simulink model "Linear_wReduced_Observer"  (R2022a)
settings: Solver=VariableStepAuto  StartTime=0.16733  StopTime=3000.0185  RelTol=1e-3
undefined symbols (not defined in the file): A_HD, A_platform, B_HD, B_platform, C_HD, C_platform, HD_FOP
settings Model: Creator=ianam  LastModifiedBy=ianam
settings DataIOCC: InitialState=IC  LoadInitialState=on
settings DebuggingCC: UnderSpecifiedDataTypeMsg=error  UnderSpecifiedDimensionMsg=error

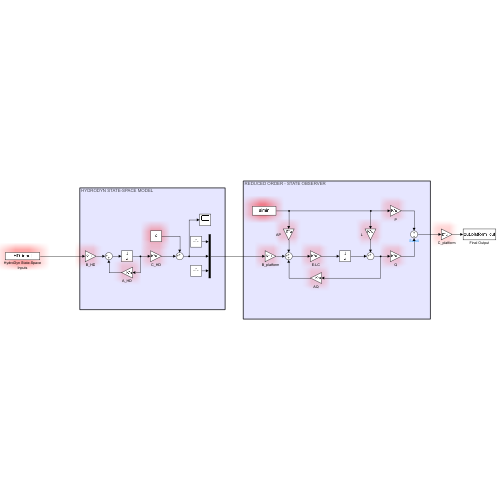
[thumbnail: Simulink's stored preview of the top-level diagram]
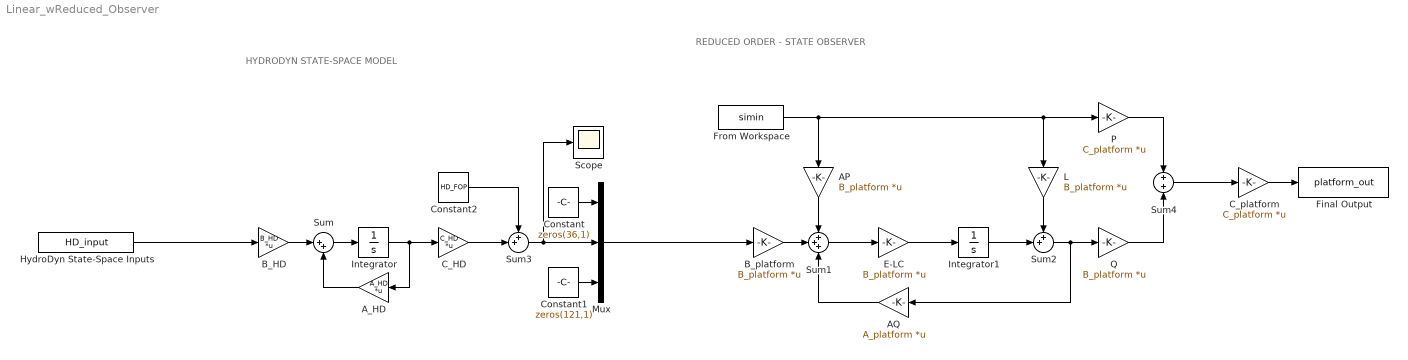
== system Linear_wReduced_Observer ==
  note: HYDRODYN STATE-SPACE MODEL
  note: REDUCED ORDER - STATE OBSERVER
  AP : Gain  Gain=B_platform  Multiplication=Matrix(K*u)
  AQ : Gain  Gain=A_platform  Multiplication=Matrix(K*u)
  A_HD : Gain  Gain=A_HD  Multiplication=Matrix(K*u)
  B_HD : Gain  Gain=B_HD  Multiplication=Matrix(K*u)
  B_platform : Gain  Gain=B_platform  Multiplication=Matrix(K*u)
  C_HD : Gain  Gain=C_HD  Multiplication=Matrix(K*u)
  C_platform : Gain  Gain=C_platform  Multiplication=Matrix(K*u)
  Constant : Constant  Value=zeros(36,1)
  Constant1 : Constant  Value=zeros(121,1)
  Constant2 : Constant  Value=HD_FOP
  E-LC : Gain  Gain=B_platform  Multiplication=Matrix(K*u)
  Final Output : ToWorkspace  VariableName=platform_out  SaveFormat=Timeseries  SampleTime=-1
  From Workspace : FromWorkspace  VariableName=simin
  HydroDyn State-Space Inputs : FromWorkspace  VariableName=HD_input
  Integrator : Integrator
  Integrator1 : Integrator
  L : Gain  Gain=B_platform  Multiplication=Matrix(K*u)
  Mux : Mux  Inputs=3
  P : Gain  Gain=C_platform  Multiplication=Matrix(K*u)
  Q : Gain  Gain=B_platform  Multiplication=Matrix(K*u)
  Scope : Scope
  Sum : Sum  Inputs=|++
  Sum1 : Sum  Inputs=+++
  Sum2 : Sum  Inputs=++|
  Sum3 : Sum  Inputs=++|
  Sum4 : Sum  Inputs=+|+
  wires:
  Sum/1 -> Integrator/1
  Integrator/1 -> C_HD/1, A_HD/1
  A_HD/1 -> Sum/2
  B_HD/1 -> Sum/1
  HydroDyn State-Space Inputs/1 -> B_HD/1
  Constant/1 -> Mux/1
  Constant1/1 -> Mux/3
  Mux/1 -> B_platform/1
  C_HD/1 -> Sum3/2
  Sum3/1 -> Scope/1, Mux/2
  Constant2/1 -> Sum3/1
  B_platform/1 -> Sum1/2
  Sum1/1 -> E-LC/1
  AP/1 -> Sum1/1
  AQ/1 -> Sum1/3
  E-LC/1 -> Integrator1/1
  Integrator1/1 -> Sum2/2
  L/1 -> Sum2/1
  Sum2/1 -> AQ/1, Q/1
  Q/1 -> Sum4/2
  P/1 -> Sum4/1
  From Workspace/1 -> L/1, P/1, AP/1
  Sum4/1 -> C_platform/1
  C_platform/1 -> Final Output/1
